simulink model "converter1_basic_test_r2024a"  (R2024a)
settings: Solver=daessc  StartTime=0  StopTime=0.4  MaxStep=1e-6  RelTol=1e-4
model workspace (MAT data in the model file):
  Fout_Hz = 50
  LoadEnable = 1
  Rphase = 9.23760430703
libraries: fl_lib x21, nesl_utility x14
settings Model: Creator=chidan  LastModifiedBy=chidan

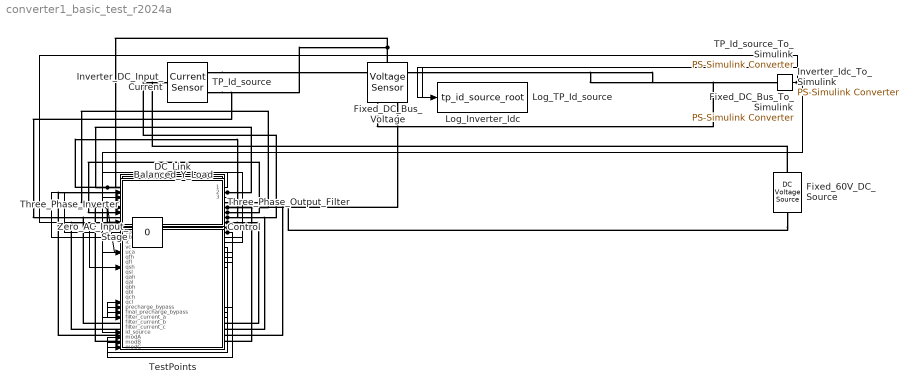
== system converter1_basic_test_r2024a ==
  Balanced_Y_Load : Subsystem
  Control : Subsystem  ReferencedSubsystem=converter1_control_r2024a
  DC_Link : Subsystem
  Fixed_60V_DC_Source : fl_lib/Electrical/Electrical Sources/DC Voltage Source  v0=60 V
  Fixed_DC_Bus_To_Simulink : nesl_utility/PS-Simulink Converter  PhysicalDomain=network_engine_domain  SubClassName=ps_output  LeftPortType=input  RightPortType=output  PseudoPeriodic=off  Frequencies=[]  VectorFormat=inherit  Unit=V  AffineConversion=off
  Fixed_DC_Bus_Voltage : fl_lib/Electrical/Electrical Sensors/Voltage Sensor
  Inverter_DC_Input_Current : fl_lib/Electrical/Electrical Sensors/Current Sensor
  Inverter_Idc_To_Simulink : nesl_utility/PS-Simulink Converter  PhysicalDomain=network_engine_domain  SubClassName=ps_output  LeftPortType=input  RightPortType=output  PseudoPeriodic=off  Frequencies=[]  VectorFormat=inherit  Unit=A  AffineConversion=off
  Log_Inverter_Idc : ToWorkspace  VariableName=acac_idc_inverter  SaveFormat=Timeseries  SampleTime=-1
  Log_TP_Id_source : ToWorkspace  VariableName=tp_id_source_root  SaveFormat=Timeseries  SampleTime=-1
  TP_Id_source : fl_lib/Electrical/Electrical Sensors/Current Sensor
  TP_Id_source_To_Simulink : nesl_utility/PS-Simulink Converter  PhysicalDomain=network_engine_domain  SubClassName=ps_output  LeftPortType=input  RightPortType=output  PseudoPeriodic=off  Frequencies=[]  VectorFormat=inherit  Unit=inherit  AffineConversion=off
  TestPoints : Subsystem
  Three_Phase_Inverter : Subsystem  ReferencedSubsystem=converter1_inverter_r2024a
  Three_Phase_Output_Filter : Subsystem  ReferencedSubsystem=converter1_filter_r2024a
  Zero_AC_Input_Stage : Constant  Value=0
  wires:
  Control/1 -> TestPoints/15(qfh)
  Control/2 -> TestPoints/16(qfl)
  Control/3 -> TestPoints/17(qsh)
  Control/4 -> TestPoints/18(qsl)
  Control/5 -> Three_Phase_Inverter/1, TestPoints/19(qah)
  Control/6 -> Three_Phase_Inverter/2, TestPoints/20(qal)
  Control/7 -> Three_Phase_Inverter/3, TestPoints/21(qbh)
  Control/8 -> Three_Phase_Inverter/4, TestPoints/22(qbl)
  Control/9 -> Three_Phase_Inverter/5, TestPoints/23(qch)
  Control/10 -> Three_Phase_Inverter/6, TestPoints/24(qcl)
  Balanced_Y_Load/2(Va) -> Control/4, TestPoints/7(va)
  Control/11 -> TestPoints/4(pfc_duty)
  Control/12 -> TestPoints/5(inverter_modulation)
  Balanced_Y_Load/1(Ia) -> TestPoints/6(ia)
  Balanced_Y_Load/3(Uab) -> TestPoints/8(uab)
  Balanced_Y_Load/4(Ib) -> TestPoints/9(ib)
  Balanced_Y_Load/5(Vb) -> TestPoints/10(vb), Control/5
  Balanced_Y_Load/6(Ubc) -> TestPoints/11(ubc)
  Balanced_Y_Load/7(Ic) -> TestPoints/12(ic)
  Balanced_Y_Load/8(Vc) -> TestPoints/13(vc), Control/6
  Balanced_Y_Load/9(Uca) -> TestPoints/14(uca)
  Control/13 -> TestPoints/25(precharge_bypass)
  Control/14 -> TestPoints/26(final_precharge_bypass)
  Inverter_Idc_To_Simulink/1 -> Log_Inverter_Idc/1
  Fixed_DC_Bus_To_Simulink/1 -> Control/3, TestPoints/3(vdc)
  Zero_AC_Input_Stage/1 -> Control/1, Control/2, TestPoints/1(vin), TestPoints/2(iin)
  TP_Id_source_To_Simulink/1 -> Log_TP_Id_source/1, TestPoints/30(id_source)
  Three_Phase_Output_Filter/1 -> TestPoints/27(filter_current_a)
  Three_Phase_Output_Filter/2 -> TestPoints/28(filter_current_b)
  Three_Phase_Output_Filter/3 -> TestPoints/29(filter_current_c)
  Control/15 -> TestPoints/31(modA)
  Control/16 -> TestPoints/32(modB)
  Control/17 -> TestPoints/33(modC)
  connections:
  Three_Phase_Inverter/RConn1 -- Three_Phase_Output_Filter/LConn1
  Three_Phase_Inverter/RConn2 -- Three_Phase_Output_Filter/LConn2
  Three_Phase_Inverter/RConn3 -- Three_Phase_Output_Filter/LConn3
  Three_Phase_Output_Filter/RConn1 -- Balanced_Y_Load/LConn1
  Three_Phase_Output_Filter/RConn2 -- Balanced_Y_Load/LConn2
  Three_Phase_Output_Filter/RConn3 -- Balanced_Y_Load/LConn3
  Three_Phase_Output_Filter/RConn4 -- Balanced_Y_Load/LConn4
  Inverter_DC_Input_Current/RConn2 -- Three_Phase_Inverter/LConn1
  Inverter_DC_Input_Current/RConn1 -- Inverter_Idc_To_Simulink/LConn1
  Inverter_DC_Input_Current/LConn1 -- DC_Link/LConn1 -- Fixed_DC_Bus_Voltage/LConn1 -- TP_Id_source/RConn2
  Three_Phase_Inverter/LConn2 -- Fixed_60V_DC_Source/RConn1 -- DC_Link/LConn2 -- Fixed_DC_Bus_Voltage/RConn2
  Fixed_DC_Bus_Voltage/RConn1 -- Fixed_DC_Bus_To_Simulink/LConn1
  Fixed_60V_DC_Source/LConn1 -- TP_Id_source/LConn1
  TP_Id_source/RConn1 -- TP_Id_source_To_Simulink/LConn1

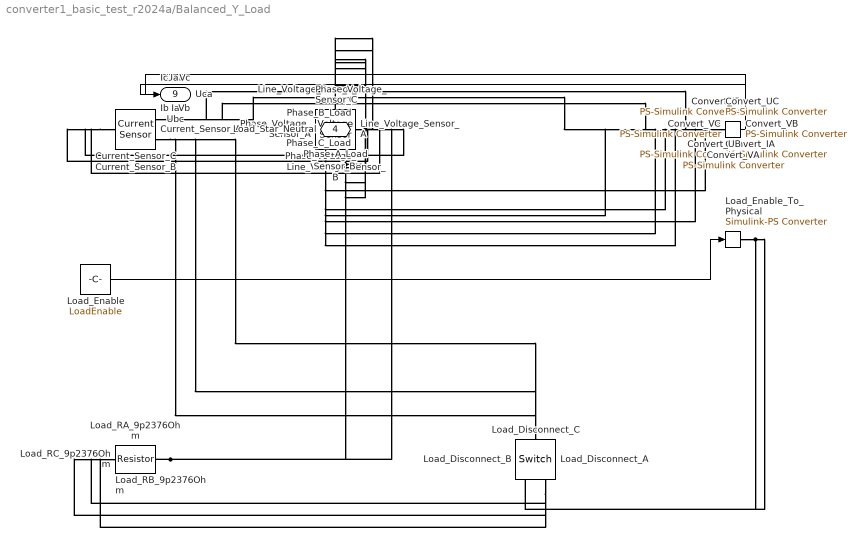
== system converter1_basic_test_r2024a/Balanced_Y_Load ==
  Convert_IA : nesl_utility/PS-Simulink Converter  PhysicalDomain=network_engine_domain  SubClassName=ps_output  LeftPortType=input  RightPortType=output  PseudoPeriodic=off  Frequencies=[]  VectorFormat=inherit  Unit=inherit  AffineConversion=off
  Convert_IB : nesl_utility/PS-Simulink Converter  PhysicalDomain=network_engine_domain  SubClassName=ps_output  LeftPortType=input  RightPortType=output  PseudoPeriodic=off  Frequencies=[]  VectorFormat=inherit  Unit=inherit  AffineConversion=off
  Convert_IC : nesl_utility/PS-Simulink Converter  PhysicalDomain=network_engine_domain  SubClassName=ps_output  LeftPortType=input  RightPortType=output  PseudoPeriodic=off  Frequencies=[]  VectorFormat=inherit  Unit=inherit  AffineConversion=off
  Convert_UA : nesl_utility/PS-Simulink Converter  PhysicalDomain=network_engine_domain  SubClassName=ps_output  LeftPortType=input  RightPortType=output  PseudoPeriodic=off  Frequencies=[]  VectorFormat=inherit  Unit=inherit  AffineConversion=off
  Convert_UB : nesl_utility/PS-Simulink Converter  PhysicalDomain=network_engine_domain  SubClassName=ps_output  LeftPortType=input  RightPortType=output  PseudoPeriodic=off  Frequencies=[]  VectorFormat=inherit  Unit=inherit  AffineConversion=off
  Convert_UC : nesl_utility/PS-Simulink Converter  PhysicalDomain=network_engine_domain  SubClassName=ps_output  LeftPortType=input  RightPortType=output  PseudoPeriodic=off  Frequencies=[]  VectorFormat=inherit  Unit=inherit  AffineConversion=off
  Convert_VA : nesl_utility/PS-Simulink Converter  PhysicalDomain=network_engine_domain  SubClassName=ps_output  LeftPortType=input  RightPortType=output  PseudoPeriodic=off  Frequencies=[]  VectorFormat=inherit  Unit=inherit  AffineConversion=off
  Convert_VB : nesl_utility/PS-Simulink Converter  PhysicalDomain=network_engine_domain  SubClassName=ps_output  LeftPortType=input  RightPortType=output  PseudoPeriodic=off  Frequencies=[]  VectorFormat=inherit  Unit=inherit  AffineConversion=off
  Convert_VC : nesl_utility/PS-Simulink Converter  PhysicalDomain=network_engine_domain  SubClassName=ps_output  LeftPortType=input  RightPortType=output  PseudoPeriodic=off  Frequencies=[]  VectorFormat=inherit  Unit=inherit  AffineConversion=off
  Current_Sensor_A : fl_lib/Electrical/Electrical Sensors/Current Sensor
  Current_Sensor_B : fl_lib/Electrical/Electrical Sensors/Current Sensor
  Current_Sensor_C : fl_lib/Electrical/Electrical Sensors/Current Sensor
  Line_Voltage_Sensor_A : fl_lib/Electrical/Electrical Sensors/Voltage Sensor
  Line_Voltage_Sensor_B : fl_lib/Electrical/Electrical Sensors/Voltage Sensor
  Line_Voltage_Sensor_C : fl_lib/Electrical/Electrical Sensors/Voltage Sensor
  Load_Disconnect_A : fl_lib/Electrical/Electrical Elements/Switch  R_closed=0.001 Ohm  G_open=1e-12 1/Ohm  Threshold=0.5  i_specify=off  i_priority=None  i=0 A  i_nominal_specify=off  i_nominal_value=1  i_nominal_unit=A  v_specify=off  v_priority=None  v=0 V  v_nominal_specify=off  v_nominal_value=1  v_nominal_unit=V
  Load_Disconnect_B : fl_lib/Electrical/Electrical Elements/Switch  R_closed=0.001 Ohm  G_open=1e-12 1/Ohm  Threshold=0.5  i_specify=off  i_priority=None  i=0 A  i_nominal_specify=off  i_nominal_value=1  i_nominal_unit=A  v_specify=off  v_priority=None  v=0 V  v_nominal_specify=off  v_nominal_value=1  v_nominal_unit=V
  Load_Disconnect_C : fl_lib/Electrical/Electrical Elements/Switch  R_closed=0.001 Ohm  G_open=1e-12 1/Ohm  Threshold=0.5  i_specify=off  i_priority=None  i=0 A  i_nominal_specify=off  i_nominal_value=1  i_nominal_unit=A  v_specify=off  v_priority=None  v=0 V  v_nominal_specify=off  v_nominal_value=1  v_nominal_unit=V
  Load_Enable : Constant  Value=LoadEnable
  Load_Enable_To_Physical : nesl_utility/Simulink-PS Converter  PhysicalDomain=network_engine_domain  SubClassName=ps_input  LeftPortType=input  RightPortType=output  PseudoPeriodic=off  Frequencies=[]  NoiseDistribution=none  NoiseParameters=[]  Unit=1  AffineConversion=off  FilteringAndDerivatives=provide  SimscapeFilterOrder=1  InputFilterTimeConstant=0.001  UdotUserProvided=0
  Load_RA_9p2376Ohm : fl_lib/Electrical/Electrical Elements/Resistor  R=Rphase Ohm  i_specify=off  i_priority=None  i=0 A  i_nominal_specify=off  i_nominal_value=1  i_nominal_unit=A  v_specify=off  v_priority=None  v=0 V  v_nominal_specify=off  v_nominal_value=1  v_nominal_unit=V
  Load_RB_9p2376Ohm : fl_lib/Electrical/Electrical Elements/Resistor  R=Rphase Ohm  i_specify=off  i_priority=None  i=0 A  i_nominal_specify=off  i_nominal_value=1  i_nominal_unit=A  v_specify=off  v_priority=None  v=0 V  v_nominal_specify=off  v_nominal_value=1  v_nominal_unit=V
  Load_RC_9p2376Ohm : fl_lib/Electrical/Electrical Elements/Resistor  R=Rphase Ohm  i_specify=off  i_priority=None  i=0 A  i_nominal_specify=off  i_nominal_value=1  i_nominal_unit=A  v_specify=off  v_priority=None  v=0 V  v_nominal_specify=off  v_nominal_value=1  v_nominal_unit=V
  Phase_Voltage_Sensor_A : fl_lib/Electrical/Electrical Sensors/Voltage Sensor
  Phase_Voltage_Sensor_B : fl_lib/Electrical/Electrical Sensors/Voltage Sensor
  Phase_Voltage_Sensor_C : fl_lib/Electrical/Electrical Sensors/Voltage Sensor
  Phase_A_Load : PMIOPort  Side=Left
  Phase_B_Load : PMIOPort  Port=2  Side=Left
  Phase_C_Load : PMIOPort  Port=3  Side=Left
  Load_Star_Neutral : PMIOPort  Port=4  Side=Left
  Ia : Outport
  Va : Outport  Port=2
  Uab : Outport  Port=3
  Ib : Outport  Port=4
  Vb : Outport  Port=5
  Ubc : Outport  Port=6
  Ic : Outport  Port=7
  Vc : Outport  Port=8
  Uca : Outport  Port=9
  wires:
  Convert_IA/1 -> Ia/1
  Convert_VA/1 -> Va/1
  Convert_IB/1 -> Ib/1
  Convert_VB/1 -> Vb/1
  Convert_IC/1 -> Ic/1
  Convert_VC/1 -> Vc/1
  Convert_UA/1 -> Uab/1
  Convert_UB/1 -> Ubc/1
  Convert_UC/1 -> Uca/1
  Load_Enable/1 -> Load_Enable_To_Physical/1
  connections:
  Current_Sensor_A/LConn1 -- Phase_A_Load/RConn1 -- Phase_Voltage_Sensor_A/LConn1 -- Line_Voltage_Sensor_A/LConn1 -- Line_Voltage_Sensor_C/RConn2
  Phase_Voltage_Sensor_A/RConn2 -- Load_Star_Neutral/RConn1 -- Load_RA_9p2376Ohm/RConn1 -- Phase_Voltage_Sensor_B/RConn2 -- Phase_Voltage_Sensor_C/RConn2 -- Load_RB_9p2376Ohm/RConn1 -- Load_RC_9p2376Ohm/RConn1
  Current_Sensor_B/LConn1 -- Phase_B_Load/RConn1 -- Phase_Voltage_Sensor_B/LConn1 -- Line_Voltage_Sensor_A/RConn2 -- Line_Voltage_Sensor_B/LConn1
  Current_Sensor_C/LConn1 -- Phase_C_Load/RConn1 -- Phase_Voltage_Sensor_C/LConn1 -- Line_Voltage_Sensor_B/RConn2 -- Line_Voltage_Sensor_C/LConn1
  Current_Sensor_A/RConn1 -- Convert_IA/LConn1
  Current_Sensor_B/RConn1 -- Convert_IB/LConn1
  Current_Sensor_C/RConn1 -- Convert_IC/LConn1
  Phase_Voltage_Sensor_A/RConn1 -- Convert_VA/LConn1
  Phase_Voltage_Sensor_B/RConn1 -- Convert_VB/LConn1
  Phase_Voltage_Sensor_C/RConn1 -- Convert_VC/LConn1
  Line_Voltage_Sensor_A/RConn1 -- Convert_UA/LConn1
  Line_Voltage_Sensor_B/RConn1 -- Convert_UB/LConn1
  Line_Voltage_Sensor_C/RConn1 -- Convert_UC/LConn1
  Current_Sensor_A/RConn2 -- Load_Disconnect_A/LConn1
  Load_Disconnect_A/RConn2 -- Load_RA_9p2376Ohm/LConn1
  Current_Sensor_B/RConn2 -- Load_Disconnect_B/LConn1
  Load_Disconnect_B/RConn2 -- Load_RB_9p2376Ohm/LConn1
  Current_Sensor_C/RConn2 -- Load_Disconnect_C/LConn1
  Load_Disconnect_C/RConn2 -- Load_RC_9p2376Ohm/LConn1
  Load_Disconnect_A/RConn1 -- Load_Enable_To_Physical/RConn1 -- Load_Disconnect_B/RConn1 -- Load_Disconnect_C/RConn1

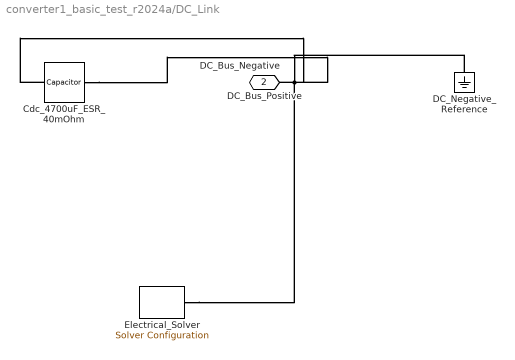
== system converter1_basic_test_r2024a/DC_Link ==
  Cdc_4700uF_ESR_40mOhm : fl_lib/Electrical/Electrical Elements/Capacitor  c=4.7e-3 F  r=0.04 Ohm  g=0 1/Ohm  i_specify=off  i_priority=None  i=0 A  i_nominal_specify=off  i_nominal_value=1  i_nominal_unit=A  v_specify=off  v_priority=None  v=0 V  v_nominal_specify=off  v_nominal_value=1  v_nominal_unit=V  vc_specify=off  vc_priority=High  vc=0 V  vc_nominal_specify=off  vc_nominal_value=1  vc_nominal_unit=V
  DC_Negative_Reference : fl_lib/Electrical/Electrical Elements/Electrical Reference
  Electrical_Solver : nesl_utility/Solver Configuration  PhysicalDomain=network_engine_domain  SubClassName=solver  LeftPortType=input  RightPortType=generic  Tones=[]  Harmonics=[]  SimulateNoise=off  Profile=off  UseLocalSampling=off  EnableSwitchedLinearOptims=on  FrequencyDomain=off  UseCCode=off  RelTol=0.001  AbsTol=0.001  MinStep=1e-09  ToWorkspace=off  RevertToSquareIcSolve=off  NumHomotopyIterations=100  PhasorMode=off  PhasorModeNumHarmonics=1  ConsistencySolver=NEWTON_XTOL_AFTER_FTOL  IndexReductionMethod=DerivativeReplacement  DoDC=off  ResidualTolerance=1e-09  ConsistencyTolSource=GLOBAL  ConsistencyAbsTol=0.001  ConsistencyRelTol=0.001  ConsistencyTolFactor=0.001  UseLocalSolver=off  LocalSolverChoice=NE_BACKWARD_EULER_ADVANCER  ResolveIndetEquations=on  FunctionEvalNumThread=1  LocalSolverSampleTime=0.001  DoFixedCost=off  MaxNonlinIter=3  MaxModeIter=2  ComputeImpulses=off  ImpulseIterations=2  LinearAlgebra=auto  LinearAlgebraNumThread=0  EquationFormulation=NE_TIME_EF  DelaysMemoryBudget=1024  AutomaticFiltering=on  FilteringTimeConstant=0.001  PartitionStorageMethod=AS_NEEDED  PartitionMemoryBudget=1024  PartitionMethod=ROBUST  MultibodyUseLocalSolver=off  MultibodyLocalSolverChoice=ODE1  MultibodyLocalSolverSampleTime=0.001
  DC_Bus_Positive : PMIOPort  Side=Left
  DC_Bus_Negative : PMIOPort  Port=2  Side=Left
  connections:
  Cdc_4700uF_ESR_40mOhm/LConn1 -- DC_Bus_Positive/RConn1
  Cdc_4700uF_ESR_40mOhm/RConn1 -- DC_Negative_Reference/LConn1 -- DC_Bus_Negative/RConn1 -- Electrical_Solver/RConn1

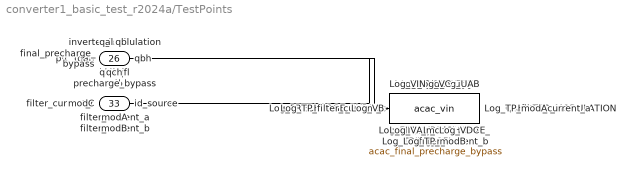
== system converter1_basic_test_r2024a/TestPoints ==
  vin : Inport
  iin : Inport  Port=2
  vdc : Inport  Port=3
  pfc_duty : Inport  Port=4
  inverter_modulation : Inport  Port=5
  ia : Inport  Port=6
  va : Inport  Port=7
  uab : Inport  Port=8
  ib : Inport  Port=9
  vb : Inport  Port=10
  ubc : Inport  Port=11
  ic : Inport  Port=12
  vc : Inport  Port=13
  uca : Inport  Port=14
  qfh : Inport  Port=15
  qfl : Inport  Port=16
  qsh : Inport  Port=17
  qsl : Inport  Port=18
  qah : Inport  Port=19
  qal : Inport  Port=20
  qbh : Inport  Port=21
  qbl : Inport  Port=22
  qch : Inport  Port=23
  qcl : Inport  Port=24
  precharge_bypass : Inport  Port=25
  final_precharge_bypass : Inport  Port=26
  filter_current_a : Inport  Port=27
  filter_current_b : Inport  Port=28
  filter_current_c : Inport  Port=29
  id_source : Inport  Port=30
  modA : Inport  Port=31
  modB : Inport  Port=32
  modC : Inport  Port=33
  Log_FINAL_PRECHARGE_BYPASS : ToWorkspace  VariableName=acac_final_precharge_bypass  SaveFormat=Timeseries  SampleTime=-1
  Log_IA : ToWorkspace  VariableName=acac_ia  SaveFormat=Timeseries  SampleTime=-1
  Log_IB : ToWorkspace  VariableName=acac_ib  SaveFormat=Timeseries  SampleTime=-1
  Log_IC : ToWorkspace  VariableName=acac_ic  SaveFormat=Timeseries  SampleTime=-1
  Log_IIN : ToWorkspace  VariableName=acac_iin  SaveFormat=Timeseries  SampleTime=-1
  Log_INVERTER_MODULATION : ToWorkspace  VariableName=acac_inverter_modulation  SaveFormat=Timeseries  SampleTime=-1
  Log_PFC_DUTY : ToWorkspace  VariableName=acac_pfc_duty  SaveFormat=Timeseries  SampleTime=-1
  Log_PRECHARGE_BYPASS : ToWorkspace  VariableName=acac_precharge_bypass  SaveFormat=Timeseries  SampleTime=-1
  Log_QAH : ToWorkspace  VariableName=acac_qah  SaveFormat=Timeseries  SampleTime=-1
  Log_QAL : ToWorkspace  VariableName=acac_qal  SaveFormat=Timeseries  SampleTime=-1
  Log_QBH : ToWorkspace  VariableName=acac_qbh  SaveFormat=Timeseries  SampleTime=-1
  Log_QBL : ToWorkspace  VariableName=acac_qbl  SaveFormat=Timeseries  SampleTime=-1
  Log_QCH : ToWorkspace  VariableName=acac_qch  SaveFormat=Timeseries  SampleTime=-1
  Log_QCL : ToWorkspace  VariableName=acac_qcl  SaveFormat=Timeseries  SampleTime=-1
  Log_QFH : ToWorkspace  VariableName=acac_qfh  SaveFormat=Timeseries  SampleTime=-1
  Log_QFL : ToWorkspace  VariableName=acac_qfl  SaveFormat=Timeseries  SampleTime=-1
  Log_QSH : ToWorkspace  VariableName=acac_qsh  SaveFormat=Timeseries  SampleTime=-1
  Log_QSL : ToWorkspace  VariableName=acac_qsl  SaveFormat=Timeseries  SampleTime=-1
  Log_TP_filter_current_a : ToWorkspace  VariableName=tp_filter_current_a  SaveFormat=Timeseries  SampleTime=-1
  Log_TP_filter_current_b : ToWorkspace  VariableName=tp_filter_current_b  SaveFormat=Timeseries  SampleTime=-1
  Log_TP_filter_current_c : ToWorkspace  VariableName=tp_filter_current_c  SaveFormat=Timeseries  SampleTime=-1
  Log_TP_id_source : ToWorkspace  VariableName=tp_id_source  SaveFormat=Timeseries  SampleTime=-1
  Log_TP_modA : ToWorkspace  VariableName=tp_moda  SaveFormat=Timeseries  SampleTime=-1
  Log_TP_modB : ToWorkspace  VariableName=tp_modb  SaveFormat=Timeseries  SampleTime=-1
  Log_TP_modC : ToWorkspace  VariableName=tp_modc  SaveFormat=Timeseries  SampleTime=-1
  Log_UAB : ToWorkspace  VariableName=acac_uab  SaveFormat=Timeseries  SampleTime=-1
  Log_UBC : ToWorkspace  VariableName=acac_ubc  SaveFormat=Timeseries  SampleTime=-1
  Log_UCA : ToWorkspace  VariableName=acac_uca  SaveFormat=Timeseries  SampleTime=-1
  Log_VA : ToWorkspace  VariableName=acac_va  SaveFormat=Timeseries  SampleTime=-1
  Log_VB : ToWorkspace  VariableName=acac_vb  SaveFormat=Timeseries  SampleTime=-1
  Log_VC : ToWorkspace  VariableName=acac_vc  SaveFormat=Timeseries  SampleTime=-1
  Log_VDC : ToWorkspace  VariableName=acac_vdc  SaveFormat=Timeseries  SampleTime=-1
  Log_VIN : ToWorkspace  VariableName=acac_vin  SaveFormat=Timeseries  SampleTime=-1
  wires:
  vin/1 -> Log_VIN/1
  iin/1 -> Log_IIN/1
  vdc/1 -> Log_VDC/1
  pfc_duty/1 -> Log_PFC_DUTY/1
  inverter_modulation/1 -> Log_INVERTER_MODULATION/1
  ia/1 -> Log_IA/1
  va/1 -> Log_VA/1
  uab/1 -> Log_UAB/1
  ib/1 -> Log_IB/1
  vb/1 -> Log_VB/1
  ubc/1 -> Log_UBC/1
  ic/1 -> Log_IC/1
  vc/1 -> Log_VC/1
  uca/1 -> Log_UCA/1
  qfh/1 -> Log_QFH/1
  qfl/1 -> Log_QFL/1
  qsh/1 -> Log_QSH/1
  qsl/1 -> Log_QSL/1
  qah/1 -> Log_QAH/1
  qal/1 -> Log_QAL/1
  qbh/1 -> Log_QBH/1
  qbl/1 -> Log_QBL/1
  qch/1 -> Log_QCH/1
  qcl/1 -> Log_QCL/1
  precharge_bypass/1 -> Log_PRECHARGE_BYPASS/1
  final_precharge_bypass/1 -> Log_FINAL_PRECHARGE_BYPASS/1
  filter_current_a/1 -> Log_TP_filter_current_a/1
  filter_current_b/1 -> Log_TP_filter_current_b/1
  filter_current_c/1 -> Log_TP_filter_current_c/1
  id_source/1 -> Log_TP_id_source/1
  modA/1 -> Log_TP_modA/1
  modB/1 -> Log_TP_modB/1
  modC/1 -> Log_TP_modC/1
